simulink model "subsampling3"  (R2021a)
settings: Solver=VariableStepAuto  StartTime=0.0  StopTime=0.1  MaxStep=1/10e6  RelTol=1e-3
values from neighbouring files (symbols this model uses):
  fnoise = 1e6    (= 1000000)    [subsampling_1.m]    (also in subsampling_2.m; subsampling_3.m = 3000000; unterabtastung_1.m; unterabtastung_2.m)
  fs = 18e3    (= 18000)    [subsampling_1.m]    (also in subsampling_2.m; subsampling_3.m = 450000; unterabtastung_1.m; unterabtastung_2.m)
  fsin = 39e3    (= 39000)    [subsampling_1.m]    (also in subsampling_2.m; subsampling_3.m = 980000; unterabtastung_1.m; unterabtastung_2.m)
undefined symbols (not defined in the file or in its folder): a, b
libraries: dspsigops x3, simulink x1, dspstat3 x1
settings Model: Creator=josef  LastModifiedBy=josef
settings SolverCC: AlgebraicLoopSolver=TrustRegion
settings DataIOCC: ReturnWorkspaceOutputs=off
settings DebuggingCC: SFMachineParentedDataDiag=warning

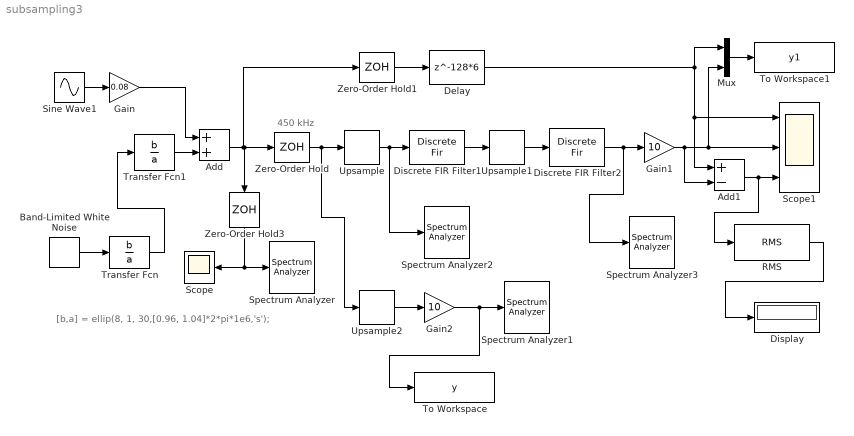
== system subsampling3 ==
  note: [b,a] = ellip(8, 1, 30,[0.96, 1.04]*2*pi*1e6,'s');
  note: 450 kHz
  Add : Sum
  Add1 : Sum  Inputs=+-
  Band-Limited White Noise : simulink/Sources/Band-Limited White Noise  Cov=1/fnoise  Ts=1/fnoise  seed=[23341]
  Delay : Delay  DelayLength=128*6
  Discrete FIR Filter1 : DiscreteFir  Coefficients=fir1(256,[0.05,0.15]*2/0.9)
  Discrete FIR Filter2 : DiscreteFir  Coefficients=fir1(256,[0.91,1.09]*2/4.5)
  Display : Display
  Gain : Gain  Gain=0.08
  Gain1 : Gain  Gain=10
  Gain2 : Gain  Gain=10
  Mux : Mux  Inputs=2
  RMS : dspstat3/RMS  run=on  directionMode=Each column  dimension=1  InputProcessing=Columns as channels (frame based)  reset_popup=None
  Scope : Scope
  Scope1 : Scope  NumInputPorts=3
  Sine Wave1 : Sin  Frequency=2*pi*fsin  SampleTime=0
  Spectrum Analyzer{,1..3} (4 alike) : SpectrumAnalyzer
  To Workspace : ToWorkspace  VariableName=y  SaveFormat=Timeseries  SampleTime=-1
  To Workspace1 : ToWorkspace  VariableName=y1  SaveFormat=Timeseries  SampleTime=-1
  Transfer Fcn : TransferFcn  Numerator=b  Denominator=a
  Transfer Fcn1 : TransferFcn  Numerator=b  Denominator=a
  Upsample : dspsigops/Upsample  N=2  phase=0  RateOptions=Allow multirate processing  ic=0  mode=Unused parameter value
  Upsample1 : dspsigops/Upsample  N=5  phase=0  RateOptions=Allow multirate processing  ic=0  mode=Unused parameter value
  Upsample2 : dspsigops/Upsample  N=10  phase=0  RateOptions=Allow multirate processing  ic=0  mode=Unused parameter value
  Zero-Order Hold : ZeroOrderHold  SampleTime=1/fs
  Zero-Order Hold1 : ZeroOrderHold  SampleTime=1/4.5e6
  Zero-Order Hold3 : ZeroOrderHold  SampleTime=1/fnoise
  wires:
  Zero-Order Hold1/1 -> Delay/1
  Delay/1 -> Add1/1, Scope1/1, Mux/1
  Band-Limited White Noise/1 -> Transfer Fcn/1
  Sine Wave1/1 -> Gain/1
  Add/1 -> Zero-Order Hold3/1, Zero-Order Hold/1, Zero-Order Hold1/1
  Zero-Order Hold3/1 -> Spectrum Analyzer/1, Scope/1
  Gain/1 -> Add/1
  Transfer Fcn/1 -> Transfer Fcn1/1
  Discrete FIR Filter1/1 -> Upsample1/1
  Gain1/1 -> Add1/2, Scope1/2, Mux/2
  Upsample1/1 -> Discrete FIR Filter2/1
  Discrete FIR Filter2/1 -> Gain1/1, Spectrum Analyzer3/1
  Zero-Order Hold/1 -> Upsample2/1, Upsample/1
  RMS/1 -> Display/1
  Upsample/1 -> Discrete FIR Filter1/1, Spectrum Analyzer2/1
  Transfer Fcn1/1 -> Add/2
  Upsample2/1 -> Gain2/1
  Gain2/1 -> To Workspace/1, Spectrum Analyzer1/1
  Add1/1 -> Scope1/3, RMS/1
  Mux/1 -> To Workspace1/1
